simulink model "pfd_overload_simulink"  (R2018a)
settings: Solver=ode45  StartTime=0.0  StopTime=0.01  FixedStep=T_ref*0.0001  RelTol=10e-5
values from neighbouring files (symbols this model uses):
  C = 10^-6    (= 1e-06)    [simulation_overload.m]
  I_p = 10^-3    (= 0.001)    [simulation_overload.m]
  initial_filter_state = v_1 - I_p*tau_1/C    [paemel_simulation.m]    (also in simulation_overload.m = 4.2)
  initial_ref_phase = 1 + tau_1/T_ref    [paemel_simulation.m]    (also in simulation_overload.m = 0.8)
  initial_vco_phase = 0    [paemel_simulation.m]    (also in simulation_overload.m)
  K_vco = 1000    [simulation_overload.m]
  omega_free = 0    [simulation_overload.m]
  R = 1000    [simulation_overload.m]
  T_ref = 10^-3    (= 0.001)    [simulation_overload.m]
  tau_1 = -0.2*T_ref    (= -0.0002)    [simulation_overload.m]
settings Model: Creator=mir  LastModifiedBy=mir

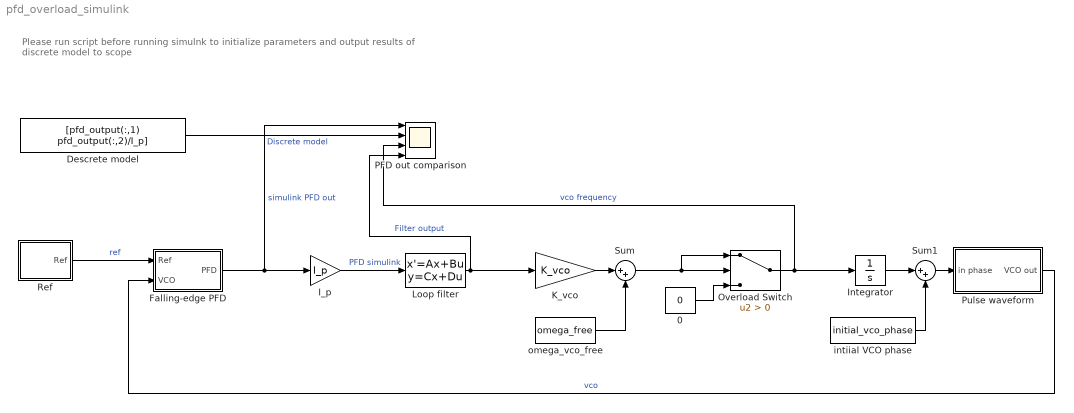
== system pfd_overload_simulink ==
  note: Please run script before running simulnk to initialize parameters
      | and output results of discrete model to scope
  0 : Constant  Value=0
  Descrete model : FromWorkspace  VariableName=[pfd_output(:,1) pfd_output(:,2)/I_p]  SampleTime=0
  Falling-edge PFD : Subsystem
  I_p : Gain  Gain=I_p
  Integrator : Integrator
  K_vco : Gain  Gain=K_vco
  Loop filter : StateSpace  A=0  B=1/C  D=R  InitialCondition=initial_filter_state
  Overload Switch : Switch  Criteria=u2 > Threshold
  PFD out comparison : Scope  NumInputPorts=4
  Pulse waveform : Subsystem
  Ref : Subsystem
  Sum : Sum  Inputs=|++
  Sum1 : Sum  Inputs=|++
  intiial VCO phase : Constant  Value=initial_vco_phase
  omega_vco_free : Constant  Value=omega_free
  wires:
  I_p/1 -> Loop filter/1  "PFD simulink"
  Falling-edge PFD/1(PFD) -> PFD out comparison/1, I_p/1  "simulink PFD out"
  omega_vco_free/1 -> Sum/2
  K_vco/1 -> Sum/1
  Loop filter/1 -> PFD out comparison/4, K_vco/1  "Filter output"
  intiial VCO phase/1 -> Sum1/2
  Pulse waveform/1(VCO out) -> Falling-edge PFD/2(VCO)  "vco"
  Ref/1(Ref) -> Falling-edge PFD/1(Ref)  "ref"
  Integrator/1 -> Sum1/1
  Sum1/1 -> Pulse waveform/1(in phase)
  Sum/1 -> Overload Switch/1, Overload Switch/2
  Overload Switch/1 -> Integrator/1, PFD out comparison/3  "vco frequency"
  0/1 -> Overload Switch/3
  Descrete model/1 -> PFD out comparison/2  "Discrete model"

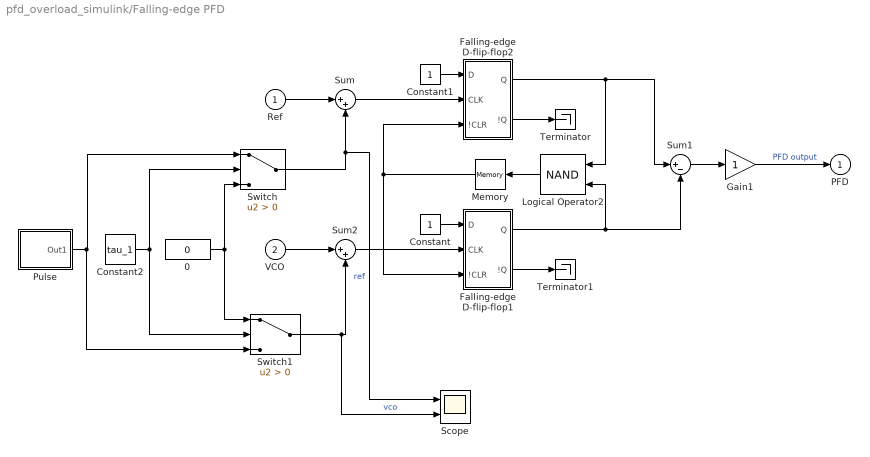
== system pfd_overload_simulink/Falling-edge PFD ==
  Ref : Inport
  VCO : Inport  Port=2
  0 : Constant  Value=0  OutDataTypeStr=boolean
  Constant : Constant  OutDataTypeStr=boolean
  Constant1 : Constant  OutDataTypeStr=boolean
  Constant2 : Constant  Value=tau_1
  Falling-edge D-flip-flop1 : Subsystem
  Falling-edge D-flip-flop2 : Subsystem
  Gain1 : Gain  SaturateOnIntegerOverflow=on  OutDataTypeStr=Inherit: Same as input  ParamDataTypeStr=Inherit: Same as input
  Logical Operator2 : Logic  Operator=NAND
  Memory : Memory
  Pulse : Subsystem
  Scope : Scope  NumInputPorts=2
  Sum : Sum  Inputs=|++
  Sum1 : Sum  Inputs=|+-  OutDataTypeStr=double  SaturateOnIntegerOverflow=on  InputSameDT=on
  Sum2 : Sum  Inputs=|++
  Switch : Switch  Criteria=u2 > Threshold
  Switch1 : Switch  Criteria=u2 > Threshold
  Terminator : Terminator
  Terminator1 : Terminator
  PFD : Outport  InitialOutput=0
  wires:
  Falling-edge D-flip-flop2/2(!Q) -> Terminator/1
  Logical Operator2/1 -> Memory/1
  Falling-edge D-flip-flop1/1(Q) -> Sum1/2, Logical Operator2/2
  Constant/1 -> Falling-edge D-flip-flop1/1(D)
  Gain1/1 -> PFD/1  "PFD output"
  Sum1/1 -> Gain1/1
  Falling-edge D-flip-flop1/2(!Q) -> Terminator1/1
  Memory/1 -> Falling-edge D-flip-flop2/3(!CLR), Falling-edge D-flip-flop1/3(!CLR)
  Constant1/1 -> Falling-edge D-flip-flop2/1(D)
  Falling-edge D-flip-flop2/1(Q) -> Logical Operator2/1, Sum1/1
  Constant2/1 -> Switch1/2, Switch/2
  Pulse/1(Out1) -> Switch1/3, Switch/1
  0/1 -> Switch1/1, Switch/3
  Ref/1 -> Sum/1
  Sum/1 -> Falling-edge D-flip-flop2/2(CLK)
  Switch/1 -> Scope/1, Sum/2  "ref"
  Sum2/1 -> Falling-edge D-flip-flop1/2(CLK)
  VCO/1 -> Sum2/1
  Switch1/1 -> Scope/2, Sum2/2  "vco"

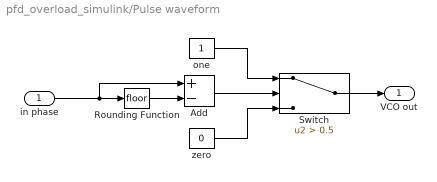
== system pfd_overload_simulink/Pulse waveform ==
  in phase : Inport
  Add : Sum  Inputs=+-
  Rounding Function : Rounding
  Switch : Switch  Criteria=u2 > Threshold  Threshold=0.5
  one : Constant
  zero : Constant  Value=0
  VCO out : Outport
  wires:
  in phase/1 -> Add/1, Rounding Function/1
  Add/1 -> Switch/2
  Rounding Function/1 -> Add/2
  one/1 -> Switch/1
  zero/1 -> Switch/3
  Switch/1 -> VCO out/1

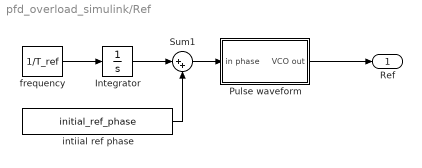
== system pfd_overload_simulink/Ref ==
  Integrator : Integrator
  Pulse waveform : Subsystem
  Sum1 : Sum  Inputs=|++
  frequency : Constant  Value=1/T_ref
  intiial ref phase : Constant  Value=initial_ref_phase
  Ref : Outport
  wires:
  intiial ref phase/1 -> Sum1/2
  Integrator/1 -> Sum1/1
  Sum1/1 -> Pulse waveform/1(in phase)
  Pulse waveform/1(VCO out) -> Ref/1
  frequency/1 -> Integrator/1

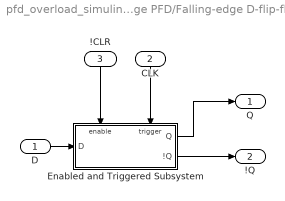
== system pfd_overload_simulink/Falling-edge PFD/Falling-edge D-flip-flop1 ==
  D : Inport
  CLK : Inport  Port=2
  !CLR : Inport  Port=3
  Enabled and Triggered Subsystem : Subsystem  TreatAsAtomicUnit=on
  Q : Outport  InitialOutput=0
  !Q : Outport  Port=2  InitialOutput=1
  wires:
  !CLR/1 -> Enabled and Triggered Subsystem/Enable
  D/1 -> Enabled and Triggered Subsystem/1(D)
  Enabled and Triggered Subsystem/1(Q) -> Q/1
  CLK/1 -> Enabled and Triggered Subsystem/Trigger
  Enabled and Triggered Subsystem/2(!Q) -> !Q/1

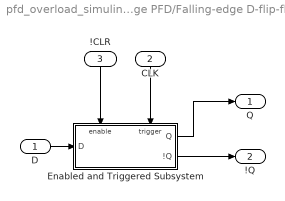
== system pfd_overload_simulink/Falling-edge PFD/Falling-edge D-flip-flop2 ==
  D : Inport
  CLK : Inport  Port=2
  !CLR : Inport  Port=3
  Enabled and Triggered Subsystem : Subsystem  TreatAsAtomicUnit=on
  Q : Outport  InitialOutput=0
  !Q : Outport  Port=2  InitialOutput=1
  wires:
  !CLR/1 -> Enabled and Triggered Subsystem/Enable
  D/1 -> Enabled and Triggered Subsystem/1(D)
  Enabled and Triggered Subsystem/1(Q) -> Q/1
  CLK/1 -> Enabled and Triggered Subsystem/Trigger
  Enabled and Triggered Subsystem/2(!Q) -> !Q/1

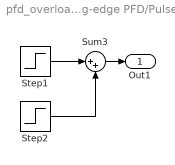
== system pfd_overload_simulink/Falling-edge PFD/Pulse ==
  Step1 : Step  Time=T_ref*0.0001  SampleTime=0
  Step2 : Step  Time=T_ref*0.0002  After=-1  SampleTime=0
  Sum3 : Sum  Inputs=|++
  Out1 : Outport
  wires:
  Sum3/1 -> Out1/1
  Step1/1 -> Sum3/1
  Step2/1 -> Sum3/2

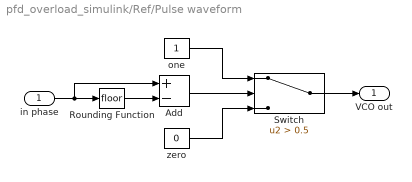
== system pfd_overload_simulink/Ref/Pulse waveform ==
  in phase : Inport
  Add : Sum  Inputs=+-
  Rounding Function : Rounding
  Switch : Switch  Criteria=u2 > Threshold  Threshold=0.5
  one : Constant
  zero : Constant  Value=0
  VCO out : Outport
  wires:
  in phase/1 -> Add/1, Rounding Function/1
  Add/1 -> Switch/2
  Rounding Function/1 -> Add/2
  one/1 -> Switch/1
  zero/1 -> Switch/3
  Switch/1 -> VCO out/1

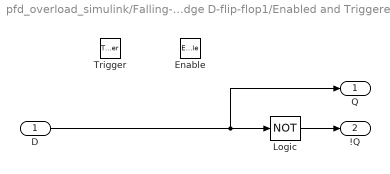
== system pfd_overload_simulink/Falling-edge PFD/Falling-edge D-flip-flop1/Enabled and Triggered Subsystem ==
  D : Inport
  Enable : EnablePort
  Trigger : TriggerPort  TriggerType=falling  VariantControl=Variant
  Logic : Logic  Operator=NOT  Inputs=1
  Q : Outport  OutputWhenDisabled=reset  InitialOutput=0
  !Q : Outport  Port=2  OutputWhenDisabled=reset  InitialOutput=1
  wires:
  D/1 -> Q/1, Logic/1
  Logic/1 -> !Q/1

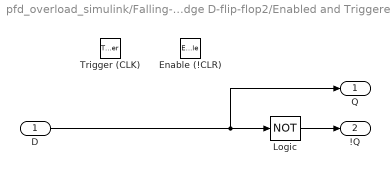
== system pfd_overload_simulink/Falling-edge PFD/Falling-edge D-flip-flop2/Enabled and Triggered Subsystem ==
  D : Inport
  Enable (!CLR) : EnablePort
  Trigger (CLK) : TriggerPort  TriggerType=falling  VariantControl=Variant
  Logic : Logic  Operator=NOT  Inputs=1
  Q : Outport  OutputWhenDisabled=reset  InitialOutput=0
  !Q : Outport  Port=2  OutputWhenDisabled=reset  InitialOutput=1
  wires:
  D/1 -> Q/1, Logic/1
  Logic/1 -> !Q/1
